simulink model "q1_a"  (R2016b)
settings: Solver=FixedStepAuto  StartTime=0.0  StopTime=50  FixedStep=0.1  RelTol=1e-3
libraries: simulink x2
settings Model: Creator=MAC  LastModifiedBy=MAC

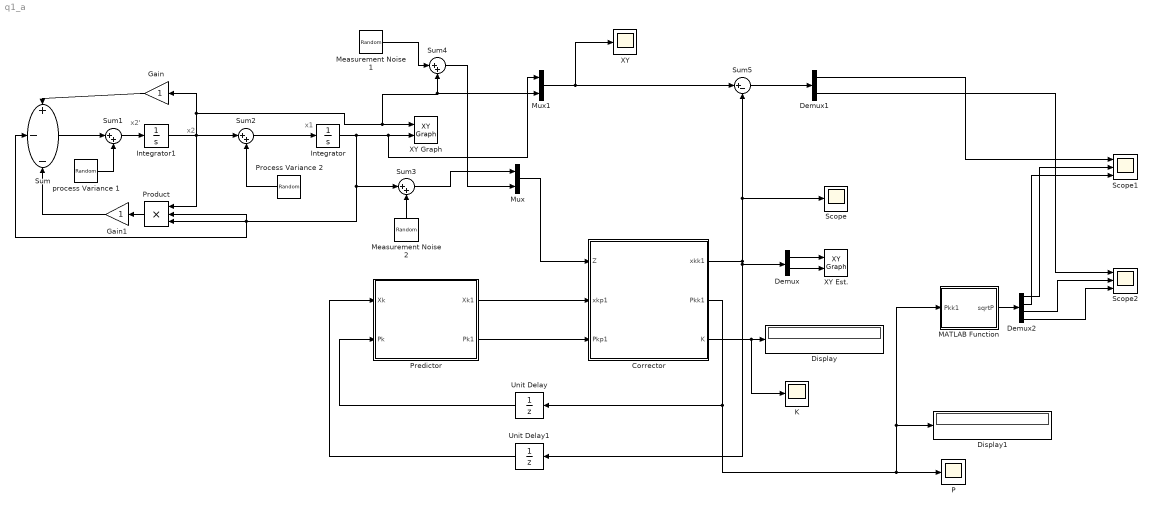
== system q1_a ==
  note: x2'
  note: x1
  note: x2
  Corrector : MATLAB Function  TreatAsAtomicUnit=on
  Demux : Demux  Outputs=2
  Demux1 : Demux  Outputs=2
  Demux2 : Demux
  Display : Display
  Display1 : Display
  Gain : Gain
  Gain1 : Gain
  Integrator : Integrator  InitialCondition=0.1
  Integrator1 : Integrator  InitialCondition=0.1
  K : Scope
  MATLAB Function : MATLAB Function  TreatAsAtomicUnit=on
  Measurement Noise 1 : RandomNumber  Variance=0.025  Seed=117  SampleTime=0.1
  "Measurement Noise 2 " : RandomNumber  Variance=0.015  Seed=113  SampleTime=0.1
  Mux : Mux  Inputs=2
  Mux1 : Mux  Inputs=2
  P : Scope
  Predictor : MATLAB Function  TreatAsAtomicUnit=on
  Process Variance 2 : RandomNumber  Variance=0.2  Seed=59  SampleTime=0.1
  Product : Product  Inputs=3
  Scope : Scope
  Scope1 : Scope  NumInputPorts=3
  Scope2 : Scope  NumInputPorts=3
  Sum : Sum  Inputs=+--
  Sum{1..4} (4 alike) : Sum  Inputs=|++
  Sum5 : Sum  Inputs=|+-
  Unit Delay : UnitDelay  InitialCondition=eye(2)  SampleTime=-1
  Unit Delay1 : UnitDelay  InitialCondition=[0.01 0.01]  SampleTime=-1
  XY : Scope
  XY Est. : simulink/Sinks/XY Graph  xmin=-3  xmax=3  ymin=-3  ymax=3  st=-1
  XY Graph : simulink/Sinks/XY Graph  xmin=-3  xmax=3  ymin=-3  ymax=3  st=-1
  process Variance 1 : RandomNumber  Variance=0.1  Seed=3  SampleTime=0.1
  wires:
  Gain/1 -> Sum/1
  Product/1 -> Gain1/1
  Gain1/1 -> Sum/3
  Sum1/1 -> Integrator1/1
  Sum/1 -> Sum1/1
  process Variance 1/1 -> Sum1/2
  Process Variance 2/1 -> Sum2/2
  Sum2/1 -> Integrator/1
  Predictor/1(Xk1) -> Corrector/2(xkp1)
  Predictor/2(Pk1) -> Corrector/3(Pkp1)
  Unit Delay/1 -> Predictor/2(Pk)
  Unit Delay1/1 -> Predictor/1(Xk)
  "Measurement Noise 2 "/1 -> Sum3/2
  Measurement Noise 1/1 -> Sum4/1
  Sum3/1 -> Mux/1
  Mux/1 -> Corrector/1(Z)
  Demux/1 -> XY Est./1
  Demux/2 -> XY Est./2
  Integrator/1 -> Mux1/1, XY Graph/2, Product/2, Sum/2, Product/3, Sum3/1
  Integrator1/1 -> Mux1/2, Sum4/2, XY Graph/1, Gain/1, Sum2/1, Product/1
  Corrector/1(xkk1) -> Demux/1, Unit Delay1/1, Scope/1, Sum5/2
  Mux1/1 -> XY/1, Sum5/1
  Sum5/1 -> Demux1/1
  Corrector/3(K) -> K/1, Display/1
  Corrector/2(Pkk1) -> MATLAB Function/1(Pkk1), Display1/1, P/1, Unit Delay/1
  Demux1/1 -> Scope1/1
  Demux1/2 -> Scope2/1
  Sum4/1 -> Mux/2
  MATLAB Function/1(sqrtP) -> Demux2/1
  Demux2/1 -> Scope1/2
  Demux2/2 -> Scope1/3
  Demux2/3 -> Scope2/2
  Demux2/4 -> Scope2/3

== matlab function q1_a/Corrector ==
  data: Z input; xkk1 output; xkp1 input; Pkp1 input; Pkk1 output; K output
function [xkk1, Pkk1, K] = corrector(Z,xkp1,Pkp1 )

xkk1=zeros(2,1);
Pkk1=zeros(2);


R=diag([0.15, 0.3]);

H=eye(2);
dh=eye(2);

K=(dh*Pkp1*(dh)'+R);
K= inv(K);
K= Pkp1*dh'* K;
Pkk1=Pkp1- (K*(dh*Pkp1*(dh)'+R)* K');
xkk1=xkp1+K*(Z-H*xkp1);

end

== matlab function q1_a/Predictor ==
  data: Xk1 output; Pk1 output; Xk input; Pk input
function [Xk1, Pk1] = predictor(Xk, Pk)
     
Xk1=zeros(2,1);
Pk1=zeros(2);

x1=Xk(1);
x2=Xk(2);
A =[0 1;
    -2*x1*x2-1 1-x1.^2];

Q = diag([4 2]);
T=0.1;
Ad=expm(A*T);
F=[-A Q;zeros(2,2) A'];
G=expm(F*T);
GLr=G(3:4,3:4);
Gur=G(1:2,3:4);
Qd=GLr'*Gur;

Xk1=Ad*Xk;
Pk1=Ad*Pk*Ad'+Qd;


end

== matlab function q1_a/MATLAB Function ==
  data: Pkk1 input; sqrtP output
function sqrtP  = sqart(Pkk1)

sqrtP=zeros(4,1);


P22=Pkk1(2,2)
sqrtP(4,1)=sqrt(abs(P22));
sqrtP(3,1)=-sqrt(abs(P22));
P11=Pkk1(1,1)
sqrtP(2,1)=sqrt(abs(P11));
sqrtP(1,1)=-sqrt(abs(P11));

end
